simulink model "pso_mppt_grid_det"  (R2024a)
settings: Solver=FixedStepDiscrete  StartTime=0.0  StopTime=2.5  RelTol=1e-3
PreLoadFcn:
  | Ts_Power=1e-6;
  | Ts_Control=100e-6;
undefined symbols (not defined in the file or in its folder): D1, Delta, sigbuilder_block
libraries: spsSeriesRLCBranchLib x5, spsMeanLib x3, spsThreePhaseTransformerTwoWindingsLib x2, spsDistributedParametersLineLib x2, spsThreePhaseParallelRLCLoadLib x2, slpidlib x2, spsabctodq0Lib x2, spsVoltageMeasurementLib x2, spsPWMGeneratorDCDCLib x1, spsThreePhaseSeriesRLCLoadLib x1, spsThreeLevelBridgeLib x1, spsThreePhaseSourceLib x1
(part 1 of 2)
Description:
  | Copyright 2008-2019 The MathWorks, Inc.
settings Model: SimulationMode=accelerator  Creator=MathWorks  LastModifiedBy=Administrator
settings SolverCC: AlgebraicLoopSolver=TrustRegion
settings DataIOCC: LimitDataPoints=on  SaveFormat=Array  SignalLoggingSaveFormat=ModelDataLogs  SignalLogging=off  DSMLogging=off  ReturnWorkspaceOutputs=off
settings OptimizationCC: ExpressionDepthLimit=2147483647  LifeSpan=inf
settings DebuggingCC: UnderspecifiedInitializationDetection=Classic  MergeDetectMultiDrivingBlocksExec=none  SolverPrmCheckMsg=warning  FcnCallInpInsideContextMsg=warning  UnconnectedInputMsg=warning  UnconnectedOutputMsg=warning  UnconnectedLineMsg=warning  StateNameClashWarn=warning  SFUnexpectedBacktrackingDiag=warning  SFNoUnconditionalDefaultTransitionDiag=warning  SFExecutionAtInitializationDiag=none  ArithmeticOperatorsInVariantConditions=warning
settings HardwareCC: ProdBitPerPointer=32  ProdBitPerSizeT=32  ProdBitPerPtrDiffT=32  ProdLargestAtomicFloat=None  ProdIntDivRoundTo=Undefined  ProdEndianess=Unspecified  ProdWordSize=32  ProdHWDeviceType=32-bit Generic
settings ModelReferenceCC: EnableRefExpFcnMdlSchedulingChecks=on  PropagateSignalLabelsOutOfModel=off
settings SFSimCC: SimUseLocalCustomCode=off  CustomCodeUndefinedFunction=UseInterfaceOnly
settings RTWCC: RTWUseLocalCustomCode=off  GPUComputeCapability=3.5
settings CodeAppCC: StateflowObjectComments=on
settings GRTTargetCC: TargetLangStandard=C89/C90 (ANSI)  CombineOutputUpdateFcns=off  GRTInterface=on
settings ConfigComp: CovMetricSettings=dw  CovSaveCumulativeToWorkspaceVar=on  CovSaveSingleToWorkspaceVar=on  CovExternalEMLEnable=off  CovSFcnEnable=off
settings SimscapeCC: SimscapeNormalizeSystem=off

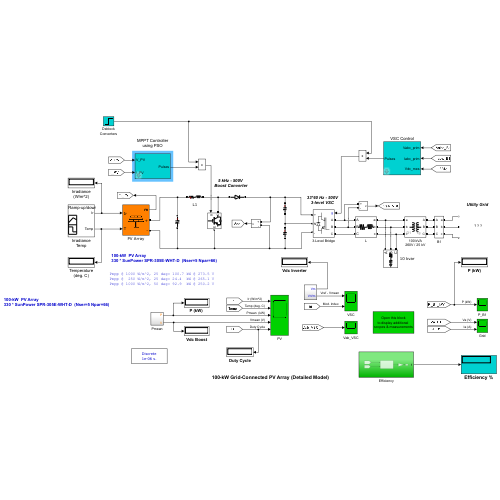
[thumbnail: Simulink's stored preview of the top-level diagram]
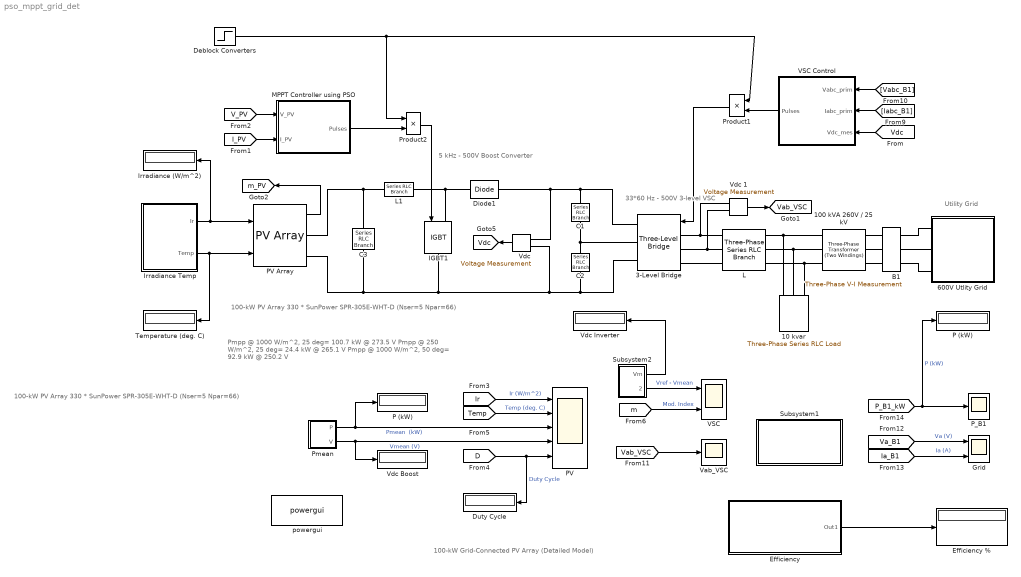
== system pso_mppt_grid_det ==
  note: 5 kHz - 500V
      | Boost Converter
  note: 33*60 Hz - 500V
      | 3-level VSC
  note: 100-kW Grid-Connected PV Array (Detailed Model)
  note: Utility Grid
  note: Pmpp @ 1000 W/m^2, 25 deg= 100.7 kW @ 273.5 V
      | Pmpp @  250 W/m^2, 25 deg= 24.4  kW @ 265.1 V
      | Pmpp @ 1000 W/m^2, 50 deg= 92.9  kW @ 250.2 V
  note: 100-kW  PV Array
      | 330 * SunPower SPR-305E-WHT-D  (Nser=5 Npar=66)
  note: 100-kW  PV Array
      | 330 * SunPower SPR-305E-WHT-D  (Nser=5 Npar=66)
  " MPPT Controller using PSO " : Subsystem  mask(Boost Control - MPPT){fc=5000, T_MPPT=200e-6, Dinit=0.5}
      mask prompts: fc "PWM switching frequency (Hz)"; T_MPPT "Time window used by MPPT control (s)"; Dinit "Initial value of duty cycle"
  10 kvar : spsThreePhaseSeriesRLCLoadLib/Three-Phase Series RLC Load  LConnTagsString=A|B|C  Configuration=Y (grounded)  NominalVoltage=240  Vabc=[1e3 1e3 1e3]  Vabcp=[1e3 1e3 1e3]  NominalFrequency=60  UnbalancedPower=off  ActivePower=10e3/100  InductivePower=0  CapacitivePower=10e3  Pabc=[10e3 9e3 11e3]  QLabc=[100 90 110]  QCabc=[100 90 110]  Pabcp=[10e3 9e3 11e3]  QLabcp=[100 90 110]  QCabcp=[100 90 110]  Measurements=None  LoadType=constant Z
  100 kVA 260V / 25 kV : spsThreePhaseTransformerTwoWindingsLib/Three-Phase Transformer (Two Windings)  Winding1Connection=Yg  Winding2Connection=Delta (D1)  CoreType=Three single-phase transformers  SetSaturation=off  Hysteresis=off  DataFile='hysteresis'  SetInitialFlux=off  Measurements=None  UNITS=pu  NominalPower=[100e3 , 60 ]  Winding1=[ 25e3 , 0.001 , 0.03 ]  Winding2=[ 260 , 0.001 , 0.03 ]  Rm=500  Lm=500  L0=0.5  Saturation=[ 0,0 ; 0.0024,1.2 ; 1.0,1.52 ]  InitialFluxes=[ 0.8 , -0.8 , 0.7 ]  BreakLoop=off  DiscreteSolver=Trapezoidal iterative  DataType=off  TransfoNumber=0
  3-Level Bridge : spsThreeLevelBridgeLib/Three-Level Bridge  Arms=3  SnubberResistance=1e6  SbubberCapacitance=inf  Device=IGBT / Diodes  Ron=0.2e-3  ForwardVoltages="[  0  0 ]"  Measurements=None
      settings: AttributesFormatString=\n  LibrarySourceBlock=sps_lib/Power Electronics/Three-Level Bridge
  600V Utlity Grid : Subsystem
      mask Display: image(imread('grid.jpg'))
  B1 : spsThreePhaseVIMeasurementLib/Three-Phase V-I Measurement  VoltageMeasurement=phase-to-ground  SetLabelV=on  LabelV=Vabc_B1  Vpu=off  VpuLL=off  CurrentMeasurement=yes  SetLabelI=on  LabelI=Iabc_B1  Ipu=off  Pbase=100e6  Vbase=500e3  OutputType=Magnitude  PhasorSimulation=off  PSBequivalent=0
  C1 : spsSeriesRLCBranchLib/Series RLC Branch  LConnTagsString=__new0  RConnTagsString=__new0  BranchType=C  Resistance=1.0  Inductance=1.0  SetiL0=off  InitialCurrent=0  Capacitance=12000e-06  Setx0=off  InitialVoltage=0  Measurements=None
  C2 : spsSeriesRLCBranchLib/Series RLC Branch  LConnTagsString=__new0  RConnTagsString=__new0  BranchType=C  Resistance=1.0  Inductance=1.0  SetiL0=off  InitialCurrent=0  Capacitance=12000e-06  Setx0=off  InitialVoltage=0  Measurements=None
  C3 : spsSeriesRLCBranchLib/Series RLC Branch  LConnTagsString=__new0  RConnTagsString=__new0  BranchType=C  Resistance=1.0  Inductance=1.0  SetiL0=off  InitialCurrent=0  Capacitance=100e-6  Setx0=off  InitialVoltage=0  Measurements=Branch voltage
  Deblock Converters : Step  Time=0.05  SampleTime=0
  Diode1 : spsDiodeLib/Diode  Ron=1e-4  Lon=0  Vf=0  IC=0  UseSnubber=off  Rs=inf  Cs=inf  Measurements=off
  Duty Cycle : Display
      settings: Format=bank  Decimation=2000
  Efficiency : Subsystem
  Efficiency % : Display
  Grid : Scope  NumInputPorts=2
  IGBT1 : spsIGBTLib/IGBT  Ron=0.001  Lon=0  Vf=0  Tf=0  Tt=0  IC=0  Rs=1e5  Cs=inf  Measurements=off
  Irradiance (W/m^2) : Display
      settings: Format=bank  Decimation=1000
  Irradiance Temp : Subsystem  Tag=STV Subsys  LoadFcn=sigbuilder_block('load');  StartFcn=sigbuilder_block('start');  StopFcn=sigbuilder_block('stop');  ClipboardFcn=sigbuilder_block('clipboard');  mask(Sigbuilder block){tuvar=[0:10]}
      mask help: Sigbuilder GUI
      mask init:
      | if ~strcmp(get_param(bdroot(gcbh),'SimulationStatus'),'stopped') tuvar = sigbuilder_block('maskInit'); end
      settings: CopyFcn=sigbuilder_block('copy');  DeleteFcn=sigbuilder_block('delete');  ModelCloseFcn=sigbuilder_block('modelClose');  PreSaveFcn=sigbuilder_block('preSave');  PauseFcn=sigbuilder_block('pause')  ContinueFcn=sigbuilder_block('continue')  NameChangeFcn=sigbuilder_block('namechange');  OpenFcn=sigbuilder_block('open',[216.75 153.75 550.5 395.25 ]);  CloseFcn=sigbuilder_block('close');
      mask Display: plot(0, 0, 100, 100,[2, 2, 32, 32, 2], [68, 8, 8, 68, 68],[32, 2], [38, 38], [32, 19, 2],[53, 60, 44], [32, 17, 17, 2],[16, 16, 31, 31]);txt = getActiveGroup(gcbh);text(2, 100, txt,'verticalAlignment', 'top');
  L : spsThreePhaseSeriesRLCBranchLib/Three-Phase Series RLC Branch  LConnTagsString=A|B|C  RConnTagsString=A|B|C  BranchType=RL  Resistance=500e-6*377/50/2  Inductance=500e-6/2  Capacitance=inf  Measurements=None
  L1 : spsSeriesRLCBranchLib/Series RLC Branch  LConnTagsString=__new0  RConnTagsString=__new0  BranchType=RL  Resistance=0.005  Inductance=5e-3  SetiL0=off  InitialCurrent=0  Capacitance=1e-6  Setx0=off  InitialVoltage=0  Measurements=None
  P (kW) : Display
      settings: Format=bank  Decimation=2000
  "P (kW) " : Display
      settings: Format=bank  Decimation=2000
  PV : Scope  NumInputPorts=5
  PV Array : spsPVArrayLib/PV Array  Npar=66  Nser=5  PlotType=array @ 1000 W/m2 & specified temperatures  S_vec="[ 1000  250 ]"  Temp_C_vec="[0 25 50  ]"  ModuleName=SunPower SPR-305E-WHT-D  PlotWhenSelected=off  Pm=305.226  Ncell=96  Voc=64.2  Isc=5.96  Vm=54.7  Im=5.58  beta_Voc_pc=-0.2727  alpha_Isc_pc=0.061745  beta_Voc=-0.17507  alpha_Isc=0.00368  IL=5.9657  I0=6.3076e-12  nI=0.94489  Rsh=393.2054  Rs=0.37428  RobustModel=off  RobustCellTemperature=313.3991  BAL=on  Tc=Tc  Tfilter=5e-5
  P_B1 : Scope
  Pmean : Subsystem
  Product1 : Product  RndMeth=Zero
  Product2 : Product  RndMeth=Zero
  Subsystem1 : Subsystem
      mask Display: disp('Open this block\nto display additional \nscopes & measurements')
  Subsystem2 : Subsystem
  Temperature (deg. C) : Display
      settings: Format=bank  Decimation=1000
  VSC : Scope  NumInputPorts=2
  VSC Control : Subsystem  mask(VSC Main Controller){nom=[ 100e3  60 ], Vnom=[ 25e3 260 ], Vnom_dc=500, RLxfo=[0.002  0.06 ], RLchoke=[2e-3  250e-6  ], K_VDCreg=[7  800], K_Ireg=[0.3 20], Ts=Ts_Control}
      mask prompts: nom "Nominal power and frequency [ Pnom(VA)  Fnom(Hz) ]:"; Vnom "Nominal primary and secondary voltages (Vrms LL) [ Vnom_prim   Vnom_sec ]:"; Vnom_dc "Nominal DC bus voltage (V):"; RLxfo "Total transformer leakage impedance (pu/Pnom) [ Rxfo  Lxf ]"; RLchoke "Choke impedance [ R(ohm) L(H) ]"; K_VDCreg "VDC regultator gains [ Kp  Ki ]:"; K_Ireg "Current regulator gains [ Kp  Ki ]:"; Ts "Sample time"
      mask init:
      | Pnom=nom(1);
      | Fnom=nom(2);
      | Vnom_prim=Vnom(1);
      | Vnom_sec=Vnom(2);
      | Zbase=Vnom_sec^2/Pnom;
      | Rtot_pu=RLxfo(1) + RLchoke(1)/Zbase;
      | Ltot_pu=RLxfo(2) + RLchoke(2)/(Zbase/(2*pi*Fnom));
      | Kp_VDCreg=K_VDCreg(1);
      | Ki_VDCreg=K_VDCreg(2);
      | Kp_Ireg=K_Ireg(1);
      | Ki_Ireg=K_Ireg(2);
      | Vdc_ref=Vnom_dc;
      | % Used to determine initial value of Boost Control (MPPT)
      | assignin('base','Vdc_ref_Inv',Vdc_ref);
  Vab_VSC : Scope
  "Vdc " : spsVoltageMeasurementLib/Voltage Measurement  Tag=PoWeRsYsTeMmEaSuReMeNt  PhasorSimulation=off  OutputType=Magnitude  PSBequivalent=0
  Vdc 1 : spsVoltageMeasurementLib/Voltage Measurement  Tag=PoWeRsYsTeMmEaSuReMeNt  PhasorSimulation=off  OutputType=Magnitude  PSBequivalent=0
  Vdc Boost : Display
      settings: Format=bank  Decimation=2000
  Vdc Inverter : Display
      settings: Format=bank  Decimation=2000
  powergui : spspowerguiLib/powergui  Priority=1  SimulationMode=Discrete  SampleTime=Ts_Power  frequency=60  Iterations=50  frequencyindice=0  Pbase=100e6  ErrMax=1e-4  UnitsV=kV  UnitsW=MW  buscounter=0  FunctionMessages=off  echomessages=off  EnableUseOfTLC=off  CurrentSourceSwitches=off  DisableSnubberDevices=off  DisableRonSwitches=off  DisableVfSwitches=off  DisplayEquations=off  AutomaticDiscreteSolvers=off  SolverType=Tustin/Backward Euler (TBE)  Interpol=off  ExternalGateDelay=off  methode=off  Ts=0  x0status=blocks  SPID=off  SwTol=0  HookPort=off  NonlinearTolerance=0  nMaxIteration=15  ContinueOnMaxIteration=off  RestoreLinks=warning  ResistiveCurrentMeasurement=off  Frange=[0:2:500]  Ylog=off  Xlog=on  ShowGrid=off  save=off  variable=ZData  structure=0  ZoomFFT=on  StartTime=0.0  cycles=1  DisplayStyle=1  fundamental=60  FreqAxis=off  MaxFrequency=1000  frequencyindicesteady=1  RmsSteady=1  display=off
  tag scope: Vab_VSC=global, Vdc=global, m_PV=global
  wires:
  "Vdc "/1 -> [Vdc]
  Product2/1 -> IGBT1/1
  " MPPT Controller using PSO "/1(Pulses) -> Product2/2
  Deblock Converters/1 -> Product2/1, Product1/1
  [Vabc_B1] -> VSC Control/1(Vabc_prim)
  [Iabc_B1] -> VSC Control/2(Iabc_prim)
  [Vdc] -> VSC Control/3(Vdc_mes)
  VSC Control/1(Pulses) -> Product1/2
  Product1/1 -> 3-Level Bridge/1
  [I_PV] -> " MPPT Controller using PSO "/2(I_PV)
  [V_PV] -> " MPPT Controller using PSO "/1(V_PV)
  Pmean/1(P) -> "P (kW) "/1, PV/3  "Pmean  (kW)"
  [m] -> VSC/2  "Mod. Index"
  Vdc 1/1 -> [Vab_VSC]
  [Vab_VSC] -> Vab_VSC/1
  [Ia_B1] -> Grid/2  "Ia (A)"
  [Va_B1] -> Grid/1  "Va (V)"
  [P_B1_kW] -> P_B1/1, P (kW)/1  "P (kW)"
  Pmean/2(V) -> Vdc Boost/1, PV/4  "Vmean (V)"
  Subsystem2/2(VrVm) -> VSC/1  "Vref - Vmean"
  Subsystem2/1(Vm) -> Vdc Inverter/1
  PV Array/1 -> [m_PV]
  Irradiance Temp/1(Ir) -> PV Array/1, Irradiance (W/m^2)/1
  Irradiance Temp/2(Temp) -> PV Array/2, Temperature (deg. C)/1
  [D] -> Duty Cycle/1, PV/5  "Duty Cycle"
  [Temp] -> PV/2  "Temp (deg. C)"
  [Ir] -> PV/1  "Ir (W/m^2)"
  Efficiency/1(Out1) -> Efficiency %/1
  connections:
  3-Level Bridge/RConn1 -- Diode1/RConn1 -- "Vdc "/LConn1 -- C1/LConn1
  L1/RConn1 -- Diode1/LConn1 -- IGBT1/LConn1
  3-Level Bridge/RConn3 -- C2/RConn1 -- "Vdc "/LConn2 -- IGBT1/RConn1 -- PV Array/RConn2 -- C3/RConn1
  3-Level Bridge/LConn1 -- L/LConn1 -- Vdc 1/LConn1
  3-Level Bridge/LConn2 -- L/LConn2 -- Vdc 1/LConn2
  3-Level Bridge/LConn3 -- L/LConn3
  L/RConn1 -- 100 kVA 260V / 25 kV/RConn1 -- 10 kvar/LConn1
  L/RConn2 -- 100 kVA 260V / 25 kV/RConn2 -- 10 kvar/LConn2
  L/RConn3 -- 100 kVA 260V / 25 kV/RConn3 -- 10 kvar/LConn3
  B1/LConn1 -- 100 kVA 260V / 25 kV/LConn1
  B1/LConn2 -- 100 kVA 260V / 25 kV/LConn2
  B1/LConn3 -- 100 kVA 260V / 25 kV/LConn3
  C2/LConn1 -- C1/RConn1 -- 3-Level Bridge/RConn2
  C3/LConn1 -- PV Array/RConn1 -- L1/LConn1
  B1/RConn2 -- 600V Utlity Grid/LConn2
  B1/RConn1 -- 600V Utlity Grid/LConn1
  B1/RConn3 -- 600V Utlity Grid/LConn3

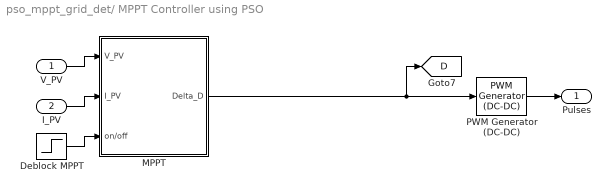
== system pso_mppt_grid_det/ MPPT Controller using PSO  ==
  V_PV : Inport
  I_PV : Inport  Port=2
  Deblock MPPT : Step  Time=0.4  SampleTime=0
  MPPT : Subsystem
  PWM Generator (DC-DC) : spsPWMGeneratorDCDCLib/PWM Generator (DC-DC)  Fsw=fc  Ts=Ts_Power
  Pulses : Outport  VectorParamsAs1DForOutWhenUnconnected=off
  tag scope: D=global
  wires:
  V_PV/1 -> MPPT/1(V_PV)
  I_PV/1 -> MPPT/2(I_PV)
  PWM Generator (DC-DC)/1 -> Pulses/1
  Deblock MPPT/1 -> MPPT/3(on/off)
  MPPT/1(Delta_D) -> PWM Generator (DC-DC)/1, [D]

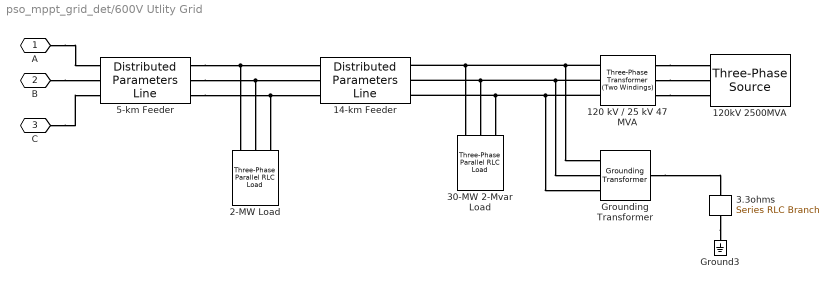
== system pso_mppt_grid_det/600V Utlity Grid ==
  120 kV / 25 kV 47 MVA : spsThreePhaseTransformerTwoWindingsLib/Three-Phase Transformer (Two Windings)  Winding1Connection=Yg  Winding2Connection=Delta (D1)  CoreType=Three single-phase transformers  SetSaturation=off  Hysteresis=off  DataFile='basic_model'  SetInitialFlux=off  Measurements=None  UNITS=pu  NominalPower=[47e6 60 ]  Winding1="[ 120e3  0.08/30   0.08 ]"  Winding2="[ 25e3  0.08/30  0.08]"  Rm=500  Lm=500  L0=0.5  Saturation="[ 0,0  ;  0.005,1.2  ;  1.0,1.4 ]"  InitialFluxes=[ 0.8 , -0.8 , 0.7 ]  BreakLoop=off  DiscreteSolver=Trapezoidal iterative  DataType=off  TransfoNumber=0
  120kV 2500MVA : spsThreePhaseSourceLib/Three-Phase Source  InternalConnection=Yg  VoltagePhases=off  Voltage=120e3  PhaseAngle=0  Voltage_phases=[25e3 25e3 25e3]/sqrt(3)  PhaseAngles_phases=[0 -120 +120]  Frequency=60  NonIdealSource=on  SpecifyImpedance=on  Resistance=0.8929  Inductance=16.58e-3  ShortCircuitLevel=2500e6  BaseVoltage=120e3  XRratio=7  BusType=swing  Pref=0  Qref=0  Prefabc=[10e3, 10e3, 10e3]  Qrefabc=[0, 0, 0]  Qmin=-inf  Qmax=inf
  14-km Feeder : spsDistributedParametersLineLib/Distributed Parameters Line  Phases=3  Length=14  Frequency=60  Resistance=[0.1153 0.413]  Inductance=[1.05e-3 3.32e-3]  Capacitance=[11.33e-009 5.01e-009]  x1=[-5.8e-05 -1.56321761301392e-09 0 0;-5.7e-05 -1.56319609439298e-09 0 0;-5.6e-05 -1.56317435360702e-09 0 0;-5.5e-05 -1.56315239065911e-09 0 0;-5.4e-05 -1.5631302055524e-09 0 0;-5.3e-05 -1.56310779829001e-09 0 0;-5.2e-05 -1.56308516887515e-09 0 0;-5.1e-05 -1.56306231731103e-09 0 0;-5e-05 -1.5630392436009e-09 0 0;-4.9e-05 -1.56301594774803e-09 -3790.73535190163 -24061.4134200248;-4.8e-05 -1.56299242975573e-09 -3781.66414358624 -24062.8407837192;-4.7e-05 -1.56296868962735e-09 -3772.59239781203 -24064.2647275473;-4.6e-05 -1.56294472736627e-09 -3763.52011586831 -24065.6852513067;-4.5e-05 -1.56292054297588e-09 -3754.44729904445 -24067.1023547955;-4.4e-05 -1.56289613645963e-09 -3745.37394862989 -24068.5160378124;-4.3e-05 -1.56287150782099e-09 -3736.30006591417 -24069.9263001563;-4.2e-05 -1.56284665706344e-09 -3727.22565218688 -24071.3331416269;-4.1e-05 -1.56282158419054e-09 -3718.15070873771 -24072.7365620243;-4e-05 -1.56279628920583e-09 -3709.0752368564 -24074.1365611489;-3.9e-05 -1.56277077211291e-09 -3699.99923783278 -24075.5331388018;-3.8e-05 -1.56274503291542e-09 -3690.92271295675 -24076.9262947845;-3.7e-05 -1.56271907161701e-09 -3681.84566351829 -24078.3160288991;-3.6e-05 -1.56269288822136e-09 -3672.76809080744 -24079.7023409479;-3.5e-05 -1.56266648273221e-09 -3663.68999611435 -24081.085230734;-3.4e-05 -1.56263985515329e-09 -3654.6113807292 -24082.4646980609;-3.3e-05 -1.56261300548841e-09 -3645.53224594227 -24083.8407427325;-3.2e-05 -1.56258593374137e-09 -3636.4525930439 -24085.2133645531;-3.1e-05 -1.56255863991601e-09 -3627.37242332452 -24086.5825633279;-3e-05 -1.56253112401623e-09 -3618.29173807463 -24087.948338862;-2.9e-05 -1.56250338604593e-09 -3609.21053858478 -24089.3106909615;-2.8e-05 -1.56247542600905e-09 -3600.12882614563 -24090.6696194327;-2.7e-05 -1.56244724390957e-09 -3591.04660204788 -24092.0251240825;-2.6e-05 -1.56241883975148e-09 -3581.96386758232 -24093.3772047183;-2.5e-05 -1.56239021353884e-09 -3572.88062403981 -24094.7258611478;-2.4e-05 -1.5623613652757e-09 -3563.79687271129 -24096.0710931794;-2.3e-05 -1.56233229496617e-09 -3554.71261488775 -24097.412900622;-2.2e-05 -1.56230300261438e-09 -3545.62785186027 -24098.7512832847;-2.1e-05 -1.56227348822449e-09 -3536.54258492 -24100.0862409775;-2e-05 -1.56224375180069e-09 -3527.45681535816 -24101.4177735105;-1.9e-05 -1.56221379334722e-09 -3518.37054446603 -24102.7458806945;-1.8e-05 -1.56218361286833e-09 -3509.28377353499 -24104.0705623409;-1.7e-05 -1.5621532103683e-09 -3500.19650385646 -24105.3918182612;-1.6e-05 -1.56212258585147e-09 -3491.10873672194 -24106.7096482678;-1.5e-05 -1.56209173932218e-09 -3482.02047342302 -24108.0240521733;-1.4e-05 -1.56206067078481e-09 -3472.93171525133 -24109.3350297909;-1.3e-05 -1.56202938024379e-09 -3463.84246349859 -24110.6425809344;-1.2e-05 -1.56199786770356e-09 -3454.75271945659 -24111.9467054178;-1.1e-05 -1.56196613316859e-09 -3445.66248441718 -24113.2474030559;-1e-05 -1.5619341766434e-09 -3436.57175967229 -24114.5446736637;-9e-06 -1.56190199813254e-09 -3427.48054651391 -24115.838517057;-8e-06 -1.56186959764056e-09 -3418.38884623411 -24117.1289330518;-7e-06 -1.56183697517209e-09 -3409.29666012501 -24118.4159214647;-6e-06 -1.56180413073174e-09 -3400.20398947883 -24119.6994821128;-5e-06 -1.5617710643242e-09 -3391.11083558782 -24120.9796148137;-4e-06 -1.56173777595416e-09 -3382.01719974435 -24122.2563193855;-3e-06 -1.56170426562636e-09 -3372.9230832408 -24123.5295956467;-2e-06 -1.56167053334555e-09 -3363.82848736966 -24124.7994434163;-1e-06 -1.56163657911652e-09 -3354.73341342347 -24126.0658625139]  x2=[-5.8e-05 -1.66978294033676e-09 0 0;-5.7e-05 -1.6697278258948e-09 0 0;-5.6e-05 -1.66967247414727e-09 0 0;-5.5e-05 -1.66961688510205e-09 0 0;-5.4e-05 -1.66956105876704e-09 0 0;-5.3e-05 -1.66950499515017e-09 0 0;-5.2e-05 -1.6694486942594e-09 0 0;-5.1e-05 -1.66939215610274e-09 0 0;-5e-05 -1.66933538068823e-09 0 0;-4.9e-05 -1.66927836802393e-09 -3379.39242591515 -24244.0512732149;-4.8e-05 -1.66922111811794e-09 -3370.25239398334 -24245.3235513048;-4.7e-05 -1.66916363097841e-09 -3361.11188306351 -24246.5923835935;-4.6e-05 -1.6691059066135e-09 -3351.97089445472 -24247.8577699007;-4.5e-05 -1.66904794503142e-09 -3342.82942945612 -24249.1197100465;-4.4e-05 -1.6689897462404e-09 -3333.6874893669 -24250.3782038516;-4.3e-05 -1.66893131024872e-09 -3324.54507548634 -24251.6332511372;-4.2e-05 -1.66887263706468e-09 -3315.40218911378 -24252.8848517248;-4.1e-05 -1.66881372669662e-09 -3306.25883154863 -24254.1330054366;-4e-05 -1.66875457915291e-09 -3297.11500409037 -24255.3777120952;-3.9e-05 -1.66869519444196e-09 -3287.97070803853 -24256.6189715237;-3.8e-05 -1.66863557257221e-09 -3278.82594469273 -24257.8567835457;-3.7e-05 -1.66857571355213e-09 -3269.68071535264 -24259.0911479852;-3.6e-05 -1.66851561739023e-09 -3260.535021318 -24260.3220646668;-3.5e-05 -1.66845528409505e-09 -3251.38886388862 -24261.5495334157;-3.4e-05 -1.66839471367516e-09 -3242.24224436437 -24262.7735540573;-3.3e-05 -1.66833390613917e-09 -3233.09516404519 -24263.9941264176;-3.2e-05 -1.66827286149574e-09 -3223.94762423108 -24265.2112503233;-3.1e-05 -1.66821157975352e-09 -3214.79962622212 -24266.4249256013;-3e-05 -1.66815006092123e-09 -3205.65117131843 -24267.6351520791;-2.9e-05 -1.66808830500762e-09 -3196.50226082022 -24268.8419295848;-2.8e-05 -1.66802631202146e-09 -3187.35289602775 -24270.0452579468;-2.7e-05 -1.66796408197155e-09 -3178.20307824136 -24271.2451369941;-2.6e-05 -1.66790161486676e-09 -3169.05280876142 -24272.4415665561;-2.5e-05 -1.66783891071595e-09 -3159.90208888841 -24273.6345464629;-2.4e-05 -1.66777596952803e-09 -3150.75091992283 -24274.8240765449;-2.3e-05 -1.66771279131195e-09 -3141.59930316529 -24276.010156633;-2.2e-05 -1.6676493760767e-09 -3132.44723991642 -24277.1927865587;-2.1e-05 -1.66758572383127e-09 -3123.29473147694 -24278.3719661539;-2e-05 -1.66752183458473e-09 -3114.14177914762 -24279.547695251;-1.9e-05 -1.66745770834614e-09 -3104.98838422931 -24280.7199736828;-1.8e-05 -1.66739334512462e-09 -3095.8345480229 -24281.8888012829;-1.7e-05 -1.66732874492933e-09 -3086.68027182936 -24283.054177885;-1.6e-05 -1.66726390776943e-09 -3077.52555694971 -24284.2161033236;-1.5e-05 -1.66719883365416e-09 -3068.37040468505 -24285.3745774335;-1.4e-05 -1.66713352259274e-09 -3059.21481633652 -24286.52960005;-1.3e-05 -1.66706797459448e-09 -3050.05879320534 -24287.6811710091;-1.2e-05 -1.66700218966867e-09 -3040.90233659279 -24288.829290147;-1.1e-05 -1.66693616782468e-09 -3031.7454478002 -24289.9739573006;-1e-05 -1.66686990907188e-09 -3022.58812812896 -24291.1151723072;-9e-06 -1.6668034134197e-09 -3013.43037888055 -24292.2529350046;-8e-06 -1.66673668087757e-09 -3004.27220135647 -24293.387245231;-7e-06 -1.666669711455e-09 -2995.11359685831 -24294.5181028254;-6e-06 -1.66660250516148e-09 -2985.95456668772 -24295.645507627;-5e-06 -1.66653506200659e-09 -2976.79511214638 -24296.7694594754;-4e-06 -1.66646738199989e-09 -2967.63523453608 -24297.8899582111;-3e-06 -1.66639946515102e-09 -2958.47493515863 -24299.0070036747;-2e-06 -1.66633131146961e-09 -2949.3142153159 -24300.1205957076;-1e-06 -1.66626292096537e-09 -2940.15307630986 -24301.2307341513]  x3=[-5.8e-05 -7.7854813363112e-12 0 0;-5.7e-05 -7.78653747717526e-12 0 0;-5.6e-05 -7.78759251139869e-12 0 0;-5.5e-05 -7.78864643883155e-12 0 0;-5.4e-05 -7.78969925932404e-12 0 0;-5.3e-05 -7.79075097272655e-12 0 0;-5.2e-05 -7.7918015788896e-12 0 0;-5.1e-05 -7.79285107766388e-12 0 0;-5e-05 -7.79389946890022e-12 0 0;-4.9e-05 -7.79494675244963e-12 -23.5442847382768 -155.68147777382;-4.8e-05 -7.79599292816327e-12 -23.4855925321581 -155.690342696941;-4.7e-05 -7.79703799589245e-12 -23.426896988213 -155.699185492992;-4.6e-05 -7.79808195548864e-12 -23.3681981147833 -155.708006160717;-4.5e-05 -7.79912480680348e-12 -23.3094959202115 -155.716804698861;-4.4e-05 -7.80016654968874e-12 -23.2507904128405 -155.725581106174;-4.3e-05 -7.80120718399639e-12 -23.1920816010137 -155.73433538141;-4.2e-05 -7.80224670957851e-12 -23.1333694930749 -155.743067523323;-4.1e-05 -7.80328512628737e-12 -23.0746540973683 -155.751777530673;-4e-05 -7.80432243397539e-12 -23.0159354222388 -155.760465402222;-3.9e-05 -7.80535863249514e-12 -22.9572134760315 -155.769131136735;-3.8e-05 -7.80639372169936e-12 -22.8984882670923 -155.777774732981;-3.7e-05 -7.80742770144093e-12 -22.8397598037672 -155.786396189731;-3.6e-05 -7.80846057157291e-12 -22.7810280944028 -155.794995505759;-3.5e-05 -7.8094923319485e-12 -22.7222931473463 -155.803572679844;-3.4e-05 -7.81052298242106e-12 -22.6635549709452 -155.812127710767;-3.3e-05 -7.81155252284412e-12 -22.6048135735475 -155.820660597312;-3.2e-05 -7.81258095307136e-12 -22.5460689635017 -155.829171338265;-3.1e-05 -7.81360827295661e-12 -22.4873211491567 -155.837659932419;-3e-05 -7.81463448235386e-12 -22.4285701388618 -155.846126378565;-2.9e-05 -7.81565958111728e-12 -22.3698159409669 -155.854570675501;-2.8e-05 -7.81668356910117e-12 -22.3110585638222 -155.862992822027;-2.7e-05 -7.81770644616e-12 -22.2522980157786 -155.871392816945;-2.6e-05 -7.81872821214839e-12 -22.1935343051872 -155.879770659062;-2.5e-05 -7.81974886692113e-12 -22.1347674403996 -155.888126347188;-2.4e-05 -7.82076841033317e-12 -22.0759974297679 -155.896459880134;-2.3e-05 -7.8217868422396e-12 -22.0172242816446 -155.904771256717;-2.2e-05 -7.82280416249568e-12 -21.9584480043827 -155.913060475754;-2.1e-05 -7.82382037095682e-12 -21.8996686063357 -155.921327536069;-2e-05 -7.82483546747861e-12 -21.8408860958573 -155.929572436485;-1.9e-05 -7.82584945191677e-12 -21.782100481302 -155.937795175832;-1.8e-05 -7.82686232412719e-12 -21.7233117710244 -155.945995752941;-1.7e-05 -7.82787408396593e-12 -21.6645199733797 -155.954174166645;-1.6e-05 -7.82888473128918e-12 -21.6057250967236 -155.962330415784;-1.5e-05 -7.82989426595331e-12 -21.5469271494121 -155.970464499197;-1.4e-05 -7.83090268781485e-12 -21.4881261398017 -155.978576415729;-1.3e-05 -7.83190999673048e-12 -21.4293220762493 -155.986666164226;-1.2e-05 -7.83291619255703e-12 -21.3705149671124 -155.994733743539;-1.1e-05 -7.8339212751515e-12 -21.3117048207488 -156.002779152522;-1e-05 -7.83492524437105e-12 -21.2528916455165 -156.010802390031;-9e-06 -7.83592810007299e-12 -21.1940754497744 -156.018803454925;-8e-06 -7.83692984211479e-12 -21.1352562418815 -156.026782346068;-7e-06 -7.83793047035408e-12 -21.0764340301974 -156.034739062326;-6e-06 -7.83892998464866e-12 -21.0176088230819 -156.042673602567;-5e-06 -7.83992838485646e-12 -20.9587806288955 -156.050585965664;-4e-06 -7.8409256708356e-12 -20.899949455999 -156.058476150493;-3e-06 -7.84192184244433e-12 -20.8411153127535 -156.066344155932;-2e-06 -7.84291689954108e-12 -20.7822782075207 -156.074189980863;-1e-06 -7.84391084198443e-12 -20.7234381486628 -156.082013624171]  x4=[-5.8e-05 4.3627087018527e-12 0 0;-5.7e-05 4.3644706519158e-12 0 0;-5.6e-05 4.36623198169028e-12 0 0;-5.5e-05 4.36799269092582e-12 0 0;-5.4e-05 4.36975277937219e-12 0 0;-5.3e-05 4.37151224677923e-12 0 0;-5.2e-05 4.3732710928969e-12 0 0;-5.1e-05 4.37502931747521e-12 0 0;-5e-05 4.37678692026428e-12 0 0;-4.9e-05 4.37854390101432e-12 -1.35581366009309 -2.15298522698308;-4.8e-05 4.38030025947562e-12 -1.35500190745795 -2.15349620368547;-4.7e-05 4.38205599539857e-12 -1.35418996224682 -2.15400687432802;-4.6e-05 4.38381110853364e-12 -1.3533778245751 -2.15451723883815;-4.5e-05 4.38556559863138e-12 -1.35256549455821 -2.15502729714334;-4.4e-05 4.38731946544244e-12 -1.3517529723116 -2.15553704917109;-4.3e-05 4.38907270871756e-12 -1.35094025795074 -2.15604649484895;-4.2e-05 4.39082532820757e-12 -1.35012735159114 -2.15655563410452;-4.1e-05 4.39257732366337e-12 -1.34931425334834 -2.15706446686544;-4e-05 4.39432869483598e-12 -1.34850096333789 -2.15757299305939;-3.9e-05 4.39607944147648e-12 -1.34768748167537 -2.1580812126141;-3.8e-05 4.39782956333604e-12 -1.34687380847641 -2.15858912545735;-3.7e-05 4.39957906016595e-12 -1.34605994385665 -2.15909673151694;-3.6e-05 4.40132793171756e-12 -1.34524588793175 -2.15960403072073;-3.5e-05 4.4030761777423e-12 -1.3444316408174 -2.16011102299662;-3.4e-05 4.40482379799173e-12 -1.34361720262934 -2.16061770827257;-3.3e-05 4.40657079221747e-12 -1.34280257348331 -2.16112408647655;-3.2e-05 4.40831716017121e-12 -1.34198775349508 -2.16163015753661;-3.1e-05 4.41006290160478e-12 -1.34117274278047 -2.16213592138081;-3e-05 4.41180801627006e-12 -1.3403575414553 -2.16264137793728;-2.9e-05 4.41355250391902e-12 -1.33954214963543 -2.16314652713417;-2.8e-05 4.41529636430375e-12 -1.33872656743675 -2.16365136889971;-2.7e-05 4.41703959717639e-12 -1.33791079497516 -2.16415590316213;-2.6e-05 4.4187822022892e-12 -1.33709483236662 -2.16466012984973;-2.5e-05 4.42052417939451e-12 -1.33627867972707 -2.16516404889085;-2.4e-05 4.42226552824476e-12 -1.33546233717253 -2.16566766021388;-2.3e-05 4.42400624859244e-12 -1.33464580481901 -2.16617096374723;-2.2e-05 4.42574634019018e-12 -1.33382908278255 -2.16667395941938;-2.1e-05 4.42748580279066e-12 -1.33301217117923 -2.16717664715884;-2e-05 4.42922463614666e-12 -1.33219507012516 -2.16767902689416;-1.9e-05 4.43096284001107e-12 -1.33137777973645 -2.16818109855396;-1.8e-05 4.43270041413683e-12 -1.33056030012928 -2.16868286206686;-1.7e-05 4.43443735827702e-12 -1.3297426314198 -2.16918431736157;-1.6e-05 4.43617367218475e-12 -1.32892477372425 -2.1696854643668;-1.5e-05 4.43790935561328e-12 -1.32810672715885 -2.17018630301135;-1.4e-05 4.43964440831591e-12 -1.32728849183986 -2.17068683322402;-1.3e-05 4.44137883004606e-12 -1.32647006788358 -2.17118705493368;-1.2e-05 4.44311262055723e-12 -1.32565145540631 -2.17168696806924;-1.1e-05 4.44484577960301e-12 -1.32483265452442 -2.17218657255965;-1e-05 4.44657830693707e-12 -1.32401366535425 -2.17268586833391;-9e-06 4.44831020231319e-12 -1.32319448801222 -2.17318485532105;-8e-06 4.45004146548523e-12 -1.32237512261474 -2.17368353345015;-7e-06 4.45177209620713e-12 -1.32155556927826 -2.17418190265035;-6e-06 4.45350209423293e-12 -1.32073582811927 -2.17467996285081;-5e-06 4.45523145931677e-12 -1.31991589925425 -2.17517771398075;-4e-06 4.45696019121285e-12 -1.31909578279976 -2.17567515596943;-3e-06 4.4586882896755e-12 -1.31827547887233 -2.17617228874615;-2e-06 4.4604157544591e-12 -1.31745498758856 -2.17666911224025;-1e-06 4.46214258531815e-12 -1.31663430906505 -2.17716562638113]  x5=5.70973484498186e-05  V1=ones(3,3)  V2=ones(3,3)  I1=ones(3,3)  I2=ones(3,3)  nHarmo=1  Measurements=None  Decoupling=off  VsMag0=0  VrMag0=0  VsAngle0=0  VrAngle0=0  IsMag0=0  IrMag0=0  IsAngle0=0  IrAngle0=0
      settings: LibrarySourceBlock=sps_lib/Power Grid Elements/Distributed Parameters Line
  2-MW Load : spsThreePhaseParallelRLCLoadLib/Three-Phase Parallel RLC Load  LConnTagsString=A|B|C  Configuration=Y (grounded)  NominalVoltage=25e3  Vabc=[1e3 1e3 1e3]  Vabcp=[1e3 1e3 1e3]  NominalFrequency=60  UnbalancedPower=off  ActivePower=2e6  InductivePower=0  CapacitivePower=0  Pabc=[10e3 9e3 11e3]  QLabc=[100 90 110]  QCabc=[100 90 110]  Pabcp=[10e3 9e3 11e3]  QLabcp=[100 90 110]  QCabcp=[100 90 110]  Measurements=None  LoadType=constant Z
  "3.3ohms " : spsSeriesRLCBranchLib/Series RLC Branch  LConnTagsString=__new0  RConnTagsString=__new0  BranchType=R  Resistance=3.3  Inductance=[]  SetiL0=off  InitialCurrent=0  Capacitance=[]  Setx0=off  InitialVoltage=0  Measurements=None
  30-MW 2-Mvar Load : spsThreePhaseParallelRLCLoadLib/Three-Phase Parallel RLC Load  LConnTagsString=A|B|C  Configuration=Y (grounded)  NominalVoltage=25e3  Vabc=[1e3 1e3 1e3]  Vabcp=[1e3 1e3 1e3]  NominalFrequency=60  UnbalancedPower=off  ActivePower=30e6  InductivePower=2e6  CapacitivePower=0  Pabc=[10e3 9e3 11e3]  QLabc=[100 90 110]  QCabc=[100 90 110]  Pabcp=[10e3 9e3 11e3]  QLabcp=[100 90 110]  QCabcp=[100 90 110]  Measurements=None  LoadType=constant Z
  5-km Feeder : spsDistributedParametersLineLib/Distributed Parameters Line  Phases=3  Length=5  Frequency=60  Resistance=[0.1153 0.413]  Inductance=[1.05e-3 3.32e-3]  Capacitance=[11.33e-009 5.01e-009]  x1=[-2.1e-05 -1.53861296656972e-09 -3537.17773129824 -24101.4118174687;-2e-05 -1.53858384697367e-09 -3528.09146196071 -24102.7435893521;-1.9e-05 -1.53855450871055e-09 -3519.00469120271 -24104.071935698;-1.8e-05 -1.53852495178452e-09 -3509.91742031565 -24105.3968563178;-1.7e-05 -1.53849517619978e-09 -3500.82965059105 -24106.7183510231;-1.6e-05 -1.53846518196056e-09 -3491.74138332049 -24108.0364196261;-1.5e-05 -1.53843496907113e-09 -3482.6526197956 -24109.3510619395;-1.4e-05 -1.53840453753579e-09 -3473.56336130811 -24110.6622777764;-1.3e-05 -1.53837388735885e-09 -3464.4736091498 -24111.9700669505;-1.2e-05 -1.53834301854467e-09 -3455.38336461252 -24113.2744292759;-1.1e-05 -1.53831193109764e-09 -3446.29262898821 -24114.5753645672;-1e-05 -1.53828062502218e-09 -3437.20140356885 -24115.8728726396;-9e-06 -1.53824910032274e-09 -3428.10968964652 -24117.1669533086;-8e-06 -1.53821735700379e-09 -3419.01748851335 -24118.4576063904;-7e-06 -1.53818539506986e-09 -3409.92480146155 -24119.7448317014;-6e-06 -1.53815321452547e-09 -3400.83162978339 -24121.0286290588;-5e-06 -1.53812081537521e-09 -3391.7379747712 -24122.3089982801;-4e-06 -1.53808819762368e-09 -3382.64383771741 -24123.5859391833;-3e-06 -1.53805536127551e-09 -3373.54921991449 -24124.8594515869;-2e-06 -1.53802230633537e-09 -3364.45412265499 -24126.12953531;-1e-06 -1.53798903280797e-09 -3355.35854723153 -24127.3961901721]  x2=[-2.1e-05 -1.56136582208046e-09 -3536.54258492 -24100.0862409775;-2e-05 -1.56133599729157e-09 -3527.45681535816 -24101.4177735105;-1.9e-05 -1.56130595060202e-09 -3518.37054446603 -24102.7458806945;-1.8e-05 -1.56127568201608e-09 -3509.28377353499 -24104.0705623409;-1.7e-05 -1.56124519153804e-09 -3500.19650385646 -24105.3918182612;-1.6e-05 -1.56121447917224e-09 -3491.10873672194 -24106.7096482678;-1.5e-05 -1.56118354492305e-09 -3482.02047342302 -24108.0240521733;-1.4e-05 -1.56115238879486e-09 -3472.93171525133 -24109.3350297909;-1.3e-05 -1.56112101079209e-09 -3463.84246349859 -24110.6425809344;-1.2e-05 -1.56108941091922e-09 -3454.75271945659 -24111.9467054178;-1.1e-05 -1.56105758918072e-09 -3445.66248441718 -24113.2474030559;-1e-05 -1.56102554558113e-09 -3436.57175967229 -24114.5446736637;-9e-06 -1.56099328012499e-09 -3427.48054651391 -24115.838517057;-8e-06 -1.5609607928169e-09 -3418.38884623411 -24117.1289330518;-7e-06 -1.56092808366147e-09 -3409.29666012501 -24118.4159214647;-6e-06 -1.56089515266334e-09 -3400.20398947883 -24119.6994821128;-5e-06 -1.5608619998272e-09 -3391.11083558782 -24120.9796148137;-4e-06 -1.56082862515776e-09 -3382.01719974435 -24122.2563193855;-3e-06 -1.56079502865977e-09 -3372.9230832408 -24123.5295956467;-2e-06 -1.56076121033799e-09 -3363.82848736966 -24124.7994434163;-1e-06 -1.56072717019724e-09 -3354.73341342347 -24126.0658625139]  x3=[-2.1e-05 -3.12573992157971e-12 -11.1569792961398 -79.1361755515044;-2e-05 -3.12693823123776e-12 -11.1271448686892 -79.1403760100002;-1.9e-05 -3.12813609648814e-12 -11.0973088598231 -79.1445652208836;-1.8e-05 -3.12933351716063e-12 -11.067471273782 -79.1487431835592;-1.7e-05 -3.13053049308504e-12 -11.0376321148064 -79.1529098974333;-1.6e-05 -3.13172702409124e-12 -11.0077913871371 -79.1570653619137;-1.5e-05 -3.13292311000919e-12 -10.9779490950151 -79.1612095764097;-1.4e-05 -3.1341187506689e-12 -10.9481052426818 -79.1653425403324;-1.3e-05 -3.13531394590044e-12 -10.9182598343785 -79.1694642530944;-1.2e-05 -3.13650869553395e-12 -10.888412874347 -79.17357471411;-1.1e-05 -3.13770299939962e-12 -10.8585643668292 -79.1776739227948;-1e-05 -3.13889685732771e-12 -10.8287143160673 -79.1817618785664;-9e-06 -3.14009026914856e-12 -10.7988627263036 -79.1858385808438;-8e-06 -3.14128323469256e-12 -10.7690096017806 -79.1899040290475;-7e-06 -3.14247575379015e-12 -10.7391549467412 -79.1939582225998;-6e-06 -3.14366782627185e-12 -10.7092987654284 -79.1980011609244;-5e-06 -3.14485945196825e-12 -10.6794410620853 -79.2020328434469;-4e-06 -3.14605063070998e-12 -10.6495818409556 -79.2060532695941;-3e-06 -3.14724136232776e-12 -10.6197211062828 -79.2100624387947;-2e-06 -3.14843164665235e-12 -10.5898588623107 -79.214060350479;-1e-06 -3.14962148351458e-12 -10.5599951132835 -79.2180470040786]  x4=[-2.1e-05 -1.9203909728374e-12 -12.5606324026108 -78.9000787577024;-2e-05 -1.9195103512461e-12 -12.5308868818072 -78.9048083977175;-1.9e-05 -1.91862945684957e-12 -12.5011395800851 -78.9095268235996;-1.8e-05 -1.917748289773e-12 -12.4713905016723 -78.9142340346782;-1.7e-05 -1.91686685014164e-12 -12.4416396507968 -78.9189300302841;-1.6e-05 -1.91598513808074e-12 -12.4118870316868 -78.92361480975;-1.5e-05 -1.91510315371563e-12 -12.3821326485709 -78.9282883724102;-1.4e-05 -1.91422089717165e-12 -12.3523765056778 -78.9329507176004;-1.3e-05 -1.91333836857419e-12 -12.3226186072364 -78.9376018446579;-1.2e-05 -1.91245556804868e-12 -12.2928589574762 -78.9422417529218;-1.1e-05 -1.91157249572057e-12 -12.2630975606266 -78.9468704417325;-1e-05 -1.91068915171539e-12 -12.2333344209173 -78.9514879104323;-9e-06 -1.90980553615867e-12 -12.2035695425784 -78.9560941583649;-8e-06 -1.90892164917599e-12 -12.17380292984 -78.9606891848758;-7e-06 -1.90803749089296e-12 -12.1440345869328 -78.9652729893117;-6e-06 -1.90715306143526e-12 -12.1142645180874 -78.9698455710212;-5e-06 -1.90626836092858e-12 -12.0844927275349 -78.9744069293546;-4e-06 -1.90538338949865e-12 -12.0547192195065 -78.9789570636634;-3e-06 -1.90449814727125e-12 -12.0249439982336 -78.9834959733011;-2e-06 -1.90361263437218e-12 -11.995167067948 -78.9880236576225;-1e-06 -1.90272685092731e-12 -11.9653884328816 -78.9925401159843]  x5=2.03919101606495e-05  V1=ones(3,3)  V2=ones(3,3)  I1=ones(3,3)  I2=ones(3,3)  nHarmo=1  Measurements=None  Decoupling=off  VsMag0=0  VrMag0=0  VsAngle0=0  VrAngle0=0  IsMag0=0  IrMag0=0  IsAngle0=0  IrAngle0=0
      settings: LibrarySourceBlock=sps_lib/Power Grid Elements/Distributed Parameters Line
  Ground3 : spsGroundLib/Ground  LConnTagsString=a
  "Grounding Transformer " : spsGroundingTransformerLib/Grounding Transformer   UNITS=pu  NominalPower="[100e6   60]"  NominalVoltage=25e3  ZeroSequenceImpedance_pu=[0.025 0.75]  MagnetizationBranch_pu=[500 500]  ZeroSequenceImpedance_SI=[0.052083 589.05]  MagnetizationBranch_SI=[1041.7 3.927e+005]  Measurements=None
      settings: LibrarySourceBlock=|
      | sps_lib/Power Grid Elements/Grounding
      | Transformer
  A : PMIOPort  Side=Left
  B : PMIOPort  Port=2  Side=Left
  C : PMIOPort  Port=3  Side=Left
  connections:
  "3.3ohms "/RConn1 -- Ground3/LConn1
  120 kV / 25 kV 47 MVA/LConn1 -- 120kV 2500MVA/RConn1
  120 kV / 25 kV 47 MVA/LConn2 -- 120kV 2500MVA/RConn2
  120 kV / 25 kV 47 MVA/LConn3 -- 120kV 2500MVA/RConn3
  120 kV / 25 kV 47 MVA/RConn1 -- "Grounding Transformer "/LConn1 -- 14-km Feeder/RConn1 -- 30-MW 2-Mvar Load/LConn1
  120 kV / 25 kV 47 MVA/RConn2 -- "Grounding Transformer "/LConn2 -- 14-km Feeder/RConn2 -- 30-MW 2-Mvar Load/LConn2
  120 kV / 25 kV 47 MVA/RConn3 -- "Grounding Transformer "/LConn3 -- 14-km Feeder/RConn3 -- 30-MW 2-Mvar Load/LConn3
  5-km Feeder/RConn1 -- 14-km Feeder/LConn1 -- 2-MW Load/LConn1
  5-km Feeder/RConn2 -- 14-km Feeder/LConn2 -- 2-MW Load/LConn2
  5-km Feeder/RConn3 -- 14-km Feeder/LConn3 -- 2-MW Load/LConn3
  A/RConn1 -- 5-km Feeder/LConn1
  B/RConn1 -- 5-km Feeder/LConn2
  C/RConn1 -- 5-km Feeder/LConn3
  "Grounding Transformer "/RConn1 -- "3.3ohms "/LConn1

== system pso_mppt_grid_det/Efficiency ==
  Gain : Gain  Gain=100
  Product : Product  Inputs=/*
  Out1 : Outport  VectorParamsAs1DForOutWhenUnconnected=off
  wires:
  [P_B1_kW] -> Product/2
  Product/1 -> Gain/1
  [Pmean_PV] -> Product/1
  Gain/1 -> Out1/1

== system pso_mppt_grid_det/Irradiance Temp ==
  Demux : Demux  Tag=STV Demux  Outputs=2
      settings: DisplayOption=none
  FromWs : FromWorkspace  Tag=STV FromWs  VariableName=tuvar
      SigBuilderData=|
      | common.afterFinalStr = 'Extrapolate'
      | common.sampleTime = '0'
      | dataSet(1).timeRange = [0 2]
      | dataSet(1).name = 'Constant Irradiance'
      | dataSet(2).timeRange = [0 2]
      | dataSet(2).name = 'Step Irradiance'
      | dataSet(3).timeRange = [0 3]
      | dataSet(3).name = 'Ramp-up/down Irradiance'
      | sbobj.Groups(1).Name = 'Constant Irradiance'
      | sbobj.Groups(1).Signals(1).Name = 'Ir'
      | sbobj.Groups(1).Signals(1).XData = [0 2]
      | sbobj.Groups(1).Signals(1).YData = [1000 1000]
      | sbobj.Groups(1).Signals(2).Name = 'Temp'
      | sbobj.Groups(1).Signals(2).XData = [0 1 1 2]
      | sbobj.Groups(1).Signals(2).YData = [0 0 1 1]
      | sbobj.Groups(1).TimeRange = [0 2]
      | sbobj.Groups(2).Name = 'Step Irradiance'
      | sbobj.Groups(2).Signals(1).Name = 'Ir'
      | sbobj.Groups(2).Signals(1).XData = [0 0.252 0.252 2]
      | sbobj.Groups(2).Signals(1).YData = [600 600 1000 1000]
      | sbobj.Groups(2).Signals(2).Name = 'Temp'
      | sbobj.Groups(2).Signals(2).XData = [0 1 1 2]
      | sbobj.Groups(2).Signals(2).YData = [0 0 1 1]
      | sbobj.Groups(2).TimeRange = [0 2]
      | sbobj.Groups(3).Name = 'Ramp-up/down Irradiance'
      | sbobj.Groups(3).Signals(1).Name = 'Ir'
      | sbobj.Groups(3).Signals(1).XData = [0 0.6 1.1 1.2 1.7 3]
      | sbobj.Groups(3).Signals(1).YData = [1000 1000 250 250 1000 1000]
      | sbobj.Groups(3).Signals(2).Name = 'Temp'
      | sbobj.Groups(3).Signals(2).XData = [0 2 2.1 3]
      | sbobj.Groups(3).Signals(2).YData = [25 25 50 50]
      | sbobj.Groups(3).TimeRange = [0 3]
  Ir : Outport  Tag=STV Outport  VectorParamsAs1DForOutWhenUnconnected=off
  Temp : Outport  Tag=STV Outport  Port=2  VectorParamsAs1DForOutWhenUnconnected=off
  wires:
  Demux/1 -> Ir/1
  FromWs/1 -> Demux/1
  Demux/2 -> Temp/1

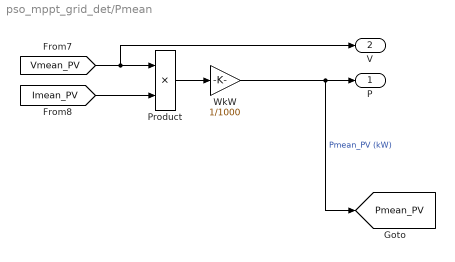
== system pso_mppt_grid_det/Pmean ==
  Product : Product  RndMeth=Zero
  WkW : Gain  Gain=1/1000
  P : Outport  VectorParamsAs1DForOutWhenUnconnected=off
  V : Outport  Port=2  VectorParamsAs1DForOutWhenUnconnected=off
  tag scope: Pmean_PV=global
  wires:
  [Vmean_PV] -> Product/1, V/1
  Product/1 -> WkW/1
  [Imean_PV] -> Product/2
  WkW/1 -> [Pmean_PV], P/1  "Pmean_PV (kW)"

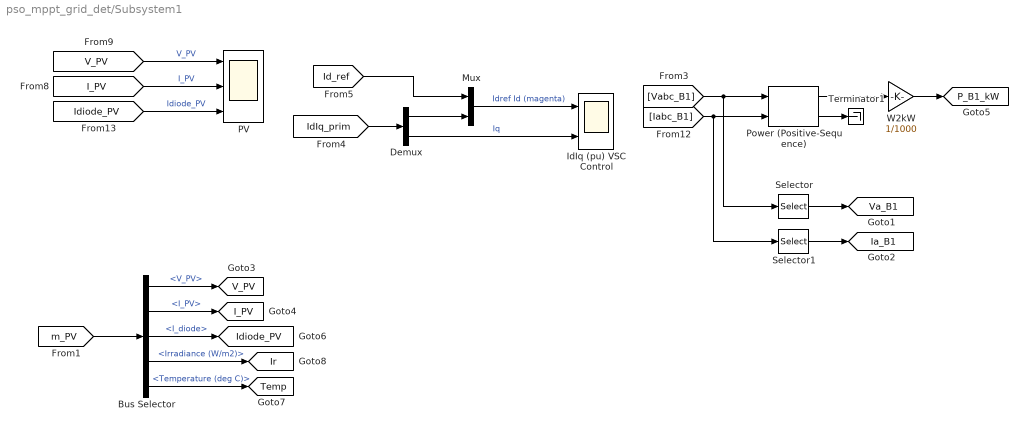
== system pso_mppt_grid_det/Subsystem1 ==
  Bus Selector : BusSelector  OutputSignals=V_PV,I_PV,I_diode,Irradiance (W/m2),Temperature (deg C)
  Demux : Demux  Outputs=2
  IdIq (pu) VSC Control : Scope  NumInputPorts=2
  Mux : Mux  Inputs=2
  PV : Scope  NumInputPorts=3
  Power (Positive-Sequence) : spsPowerPositiveSequenceLib/Power (Positive-Sequence)  Freq=60  Vinit=[0, 0]  Iinit=[0, 0]  Ts=Ts_Control
      settings: LibrarySourceBlock=|
      | sps_lib/Sensors and Measurements/Power
      | (Positive-Sequence)
  Selector : Selector  InputPortWidth=3  IndexOptions=Index vector (dialog)  Indices=[1]  OutputSizes=1
  Selector1 : Selector  InputPortWidth=3  IndexOptions=Index vector (dialog)  Indices=[1]  OutputSizes=1
  Terminator1 : Terminator
  W2kW : Gain  Gain=1/1000
  tag scope: I_PV=global, Ia_B1=global, Idiode_PV=global, Ir=global, P_B1_kW=global, Temp=global, V_PV=global, Va_B1=global
  wires:
  [Vabc_B1] -> Power (Positive-Sequence)/1, Selector/1
  [Iabc_B1] -> Power (Positive-Sequence)/2, Selector1/1
  Power (Positive-Sequence)/1 -> W2kW/1
  [IdIq_prim] -> Demux/1
  [Id_ref] -> Mux/1
  Demux/1 -> Mux/2
  Mux/1 -> IdIq (pu) VSC Control/1  "Idref Id (magenta)"
  Demux/2 -> IdIq (pu) VSC Control/2  "Iq"
  Selector/1 -> [Va_B1]
  Selector1/1 -> [Ia_B1]
  [V_PV] -> PV/1  "V_PV"
  [I_PV] -> PV/2  "I_PV"
  [Idiode_PV] -> PV/3  "Idiode_PV"
  W2kW/1 -> [P_B1_kW]
  [m_PV] -> Bus Selector/1
  Bus Selector/1 -> [V_PV]  "<V_PV>"
  Bus Selector/2 -> [I_PV]  "<I_PV>"
  Bus Selector/4 -> [Ir]  "<Irradiance (W/m2)>"
  Bus Selector/3 -> [Idiode_PV]  "<I_diode>"
  Bus Selector/5 -> [Temp]  "<Temperature (deg C)>"
  Power (Positive-Sequence)/2 -> Terminator1/1

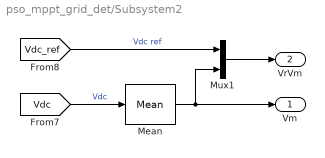
== system pso_mppt_grid_det/Subsystem2 ==
  Mean : spsMeanLib/Mean  Freq=60  Vinit=0  Ts=Ts_Control
  Mux1 : Mux  Inputs=2
  Vm : Outport  VectorParamsAs1DForOutWhenUnconnected=off
  VrVm : Outport  Port=2  VectorParamsAs1DForOutWhenUnconnected=off
  wires:
  [Vdc_ref] -> Mux1/1  "Vdc ref"
  [Vdc] -> Mean/1  "Vdc"
  Mux1/1 -> VrVm/1
  Mean/1 -> Mux1/2, Vm/1

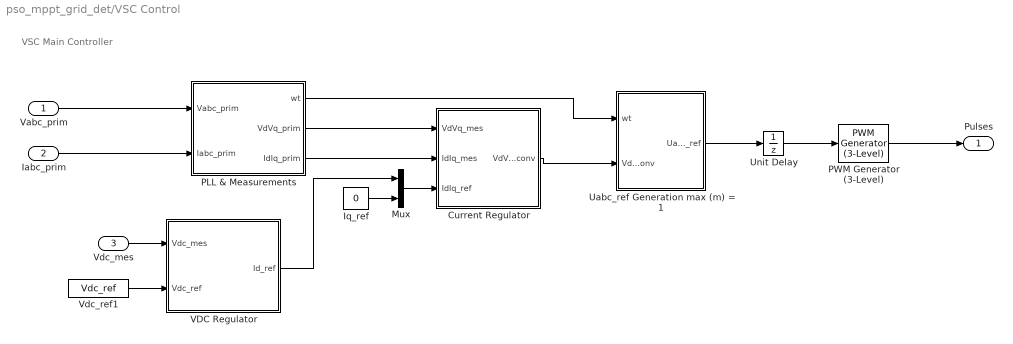
== system pso_mppt_grid_det/VSC Control ==
  note: VSC Main Controller
  Vabc_prim : Inport  PortDimensions=3
  Iabc_prim : Inport  Port=2  PortDimensions=3
  Vdc_mes : Inport  Port=3  PortDimensions=1
  Current Regulator : Subsystem
  Iq_ref : Constant  Value=0
  Mux : Mux  Inputs=2
  PLL & Measurements : Subsystem
  PWM Generator (3-Level) : spsPWMGenerator3LevelLib/PWM Generator (3-Level)  ModulatorType=Three-phase bridge (12 pulses)  ModulatorMode=Unsynchronized  nF=27  Fc=33*60  ModulatingSignals=off  m=0.8  Freq=60  Phase=0  Ts=Ts_Power
      settings: LibrarySourceBlock=|
      | sps_lib/Power Electronics/Power Electronics Control/PWM Generator
      | (3-Level)
  Uabc_ref Generation max (m) = 1 : Subsystem
  Unit Delay : UnitDelay  SampleTime=Ts_Control  HasFrameUpgradeWarning=on
  VDC Regulator : Subsystem
  Vdc_ref1 : Constant  Value=Vdc_ref
  Pulses : Outport  VectorParamsAs1DForOutWhenUnconnected=off
  wires:
  VDC Regulator/1(Id_ref) -> Mux/1
  PLL & Measurements/1(wt) -> Uabc_ref Generation max (m) = 1/1(wt)
  Current Regulator/1(VdVq_conv) -> Uabc_ref Generation max (m) = 1/2(VdVq_conv)
  Iq_ref/1 -> Mux/2
  Mux/1 -> Current Regulator/3(IdIq_ref)
  PLL & Measurements/3(IdIq_prim) -> Current Regulator/2(IdIq_mes)
  PLL & Measurements/2(VdVq_prim) -> Current Regulator/1(VdVq_mes)
  Vdc_mes/1 -> VDC Regulator/1(Vdc_mes)
  Vabc_prim/1 -> PLL & Measurements/1(Vabc_prim)
  Iabc_prim/1 -> PLL & Measurements/2(Iabc_prim)
  Unit Delay/1 -> PWM Generator (3-Level)/1
  PWM Generator (3-Level)/1 -> Pulses/1
  Uabc_ref Generation max (m) = 1/1(Uabc_ref) -> Unit Delay/1
  Vdc_ref1/1 -> VDC Regulator/2(Vdc_ref)

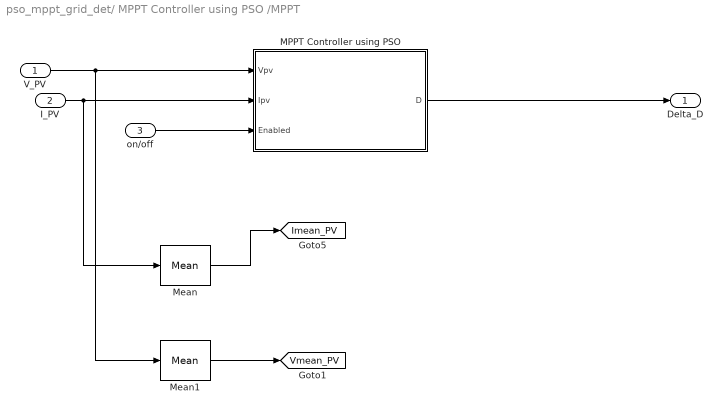
== system pso_mppt_grid_det/ MPPT Controller using PSO /MPPT ==
  V_PV : Inport
  I_PV : Inport  Port=2
  on/off : Inport  Port=3
  "MPPT Controller using PSO " : MATLAB Function  TreatAsAtomicUnit=on
  Mean : spsMeanLib/Mean  Freq=1/T_MPPT  Vinit=0  Ts=Ts_Control
  Mean1 : spsMeanLib/Mean  Freq=1/T_MPPT  Vinit=0  Ts=Ts_Control
  Delta_D : Outport  VectorParamsAs1DForOutWhenUnconnected=off
  tag scope: Imean_PV=global, Vmean_PV=global
  wires:
  Mean1/1 -> [Vmean_PV]
  Mean/1 -> [Imean_PV]
  V_PV/1 -> Mean1/1, "MPPT Controller using PSO "/1(Vpv)
  I_PV/1 -> Mean/1, "MPPT Controller using PSO "/2(Ipv)
  on/off/1 -> "MPPT Controller using PSO "/3(Enabled)
  "MPPT Controller using PSO "/1(D) -> Delta_D/1

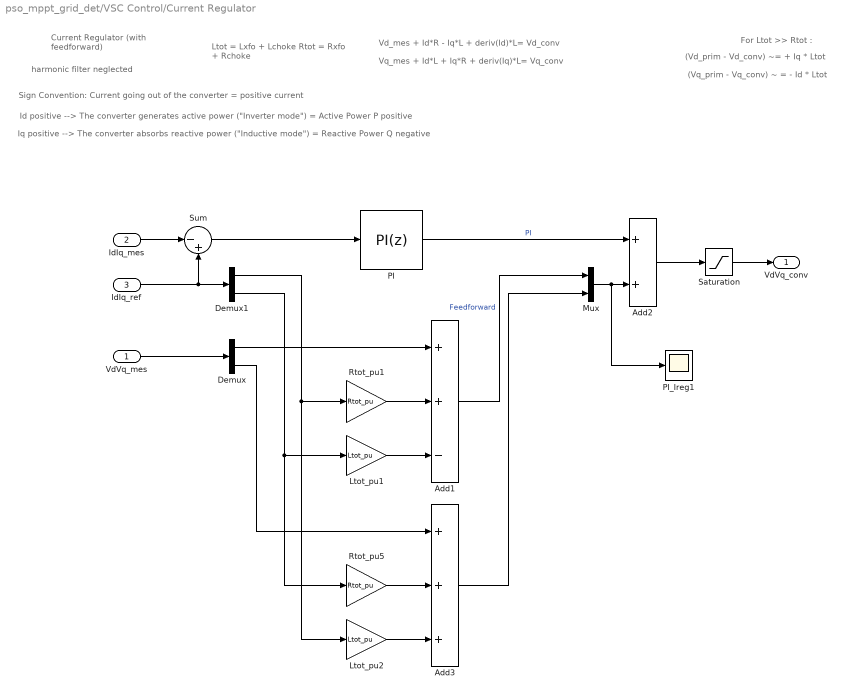
== system pso_mppt_grid_det/VSC Control/Current Regulator ==
  note: harmonic filter neglected
  note: Vd_mes + Id*R - Iq*L + deriv(Id)*L= Vd_conv
  note: Vq_mes + Id*L + Iq*R + deriv(Iq)*L= Vq_conv
  note: Current Regulator
      | (with feedforward)
  note: Sign Convention: Current going out of the converter = positive current
  note: Iq positive --> The converter absorbs reactive power ("Inductive mode") = Reactive Power Q negative
  note: Id positive --> The converter generates active power ("Inverter mode") = Active Power P positive
  note: Ltot = Lxfo + Lchoke
      | Rtot = Rxfo + Rchoke
  note: (Vd_prim - Vd_conv) ~= + Iq * Ltot
  note: (Vq_prim - Vq_conv) ~ = - Id * Ltot
  note: For Ltot >> Rtot :
  VdVq_mes : Inport  PortDimensions=2
  IdIq_mes : Inport  Port=2  PortDimensions=2
  IdIq_ref : Inport  Port=3  PortDimensions=2
  Add1 : Sum  Inputs=++-
  Add2 : Sum
  Add3 : Sum  Inputs=+++
  Demux : Demux  Outputs=2
  Demux1 : Demux  Outputs=2
  Ltot_pu1 : Gain  Gain=Ltot_pu  SaturateOnIntegerOverflow=on  OutDataTypeStr=Inherit: Same as input  ParamDataTypeStr=Inherit: Same as input
  Ltot_pu2 : Gain  Gain=Ltot_pu  SaturateOnIntegerOverflow=on  OutDataTypeStr=Inherit: Same as input  ParamDataTypeStr=Inherit: Same as input
  Mux : Mux  Inputs=2
  PI : slpidlib/PID Controller  Controller=PI  Form=Parallel  TimeDomain=Discrete-time  UseExternalTs=off  SampleTime=Ts  IntegratorMethod=Forward Euler  FilterMethod=Forward Euler  ControllerParametersSource=internal  P=Kp_Ireg  I=Ki_Ireg  UseKiTs=off  D=0  UseExternalDerivativeSource=off  N=100  UseFilter=on  TunerSelectOption=Transfer Function Based (PID Tuner App)  InitialConditionSource=internal  InitialConditionForIntegrator=0  InitialConditionForFilter=0  DifferentiatorICPrevScaledInput=0  ExternalReset=none  TrackingMode=off  Kt=1  LimitOutput=on  SatLimitsSource=internal  UpperSaturationLimit=2  LowerSaturationLimit=-2  LinearizeAsGain=off  AntiWindupMode=none  Kb=1  LimitIntegrator=off  UpperIntegratorSaturationLimit=inf  LowerIntegratorSaturationLimit=-inf  POutMin=[]  POutMax=[]  IOutMin=[]  IOutMax=[]  DOutMin=[]  DOutMax=[]  NOutMin=[]  NOutMax=[]  SumOutMin=[]  SumOutMax=[]  SaturationOutMin=[]  SaturationOutMax=[]  PParamMin=[]  PParamMax=[]  IParamMin=[]  IParamMax=[]  DParamMin=[]  DParamMax=[]  NParamMin=[]  NParamMax=[]  KbParamMin=[]  KbParamMax=[]  KtParamMin=[]  KtParamMax=[]  KbOutMin=[]  KbOutMax=[]  KtOutMin=[]  KtOutMax=[]  IntegratorOutMin=[]  IntegratorOutMax=[]  FilterOutMin=[]  FilterOutMax=[]  SumI1OutMin=[]  SumI1OutMax=[]  SumI2OutMin=[]  SumI2OutMax=[]  SumI3OutMin=[]  SumI3OutMax=[]  SumI4OutMin=[]  SumI4OutMax=[]  SumDOutMin=[]  SumDOutMax=[]  DifferentiatorOutMin=[]  DifferentiatorOutMax=[]  FilterDiffOutCoefMin=[]  FilterDiffOutCoefMax=[]  ReciprocalOutMin=[]  ReciprocalOutMax=[]  SumDenOutMin=[]  SumDenOutMax=[]  SumNumOutMin=[]  SumNumOutMax=[]  DivideOutMin=[]  DivideOutMax=[]  UdiffTsProdOutMin=[]  UdiffTsProdOutMax=[]  NTsProdOutMin=[]  NTsProdOutMax=[]  UintegralTsProdOutMin=[]  UintegralTsProdOutMax=[]  UngainTsProdOutMin=[]  UngainTsProdOutMax=[]  ClampingZeroOutDataTypeStr=Inherit: Inherit via back propagation  ClampingZeroOutMin=[]  ClampingZeroOutMax=[]  FilterDenConstantOutDataTypeStr=Inherit: Inherit via back propagation  FilterDenConstantOutMin=[]  FilterDenConstantOutMax=[]  PCopyOutDataTypeStr=Inherit: Inherit via back propagation  PCopyOutMin=[]  PCopyOutMax=[]  NCopyOutDataTypeStr=Inherit: Inherit via back propagation  NCopyOutMin=[]  NCopyOutMax=[]  IntegratorContinuousStateAttributes=''  IntegratorStateMustResolveToSignalObject=off  IntegratorRTWStateStorageClass=Auto  FilterContinuousStateAttributes=''  FilterStateMustResolveToSignalObject=off  FilterRTWStateStorageClass=Auto  ParallelPVariant=InternalParameters  IdealPVariant=Disabled  IVariant=InternalParameters  DVariant=Disabled  IntegratorVariant=Discrete  SatVariant=Enabled  AWVariant=Passthrough  PCopyVariant=Disabled  TRVariant=Disabled  FdbkBlocksVariant=Forward  IdealPFdbkVariant=Disabled  SatFdbkVariant=Disabled  DerivativeFilterVariant=Disabled  NVariant=Disabled  NCopyVariant=Disabled_SignalSpec  FilterICVariant=Disabled  IntegratorICVariant=InternalICs  ExternalResetVariant=Disabled  TRSumVariant=Passthrough  SumFdbkVariant=Disabled  SumVariant=Sum_PI  TsampFilterVariant=InternalTs  TsampNgainVariant=Passthrough  TsampIntegralVariant=Disabled_SignalSpec  ExternalSaturationOutDataTypeStr=Inherit: Same as second input  DerivativeSourceVariant=Disabled
  PI_Ireg1 : Scope
  Rtot_pu1 : Gain  Gain=Rtot_pu  SaturateOnIntegerOverflow=on  OutDataTypeStr=Inherit: Same as input  ParamDataTypeStr=Inherit: Same as input
  Rtot_pu5 : Gain  Gain=Rtot_pu  SaturateOnIntegerOverflow=on  OutDataTypeStr=Inherit: Same as input  ParamDataTypeStr=Inherit: Same as input
  Saturation : Saturate  UpperLimit=2  LowerLimit=-2
  Sum : Sum  Inputs=|-+
  VdVq_conv : Outport  VectorParamsAs1DForOutWhenUnconnected=off
  wires:
  Mux/1 -> PI_Ireg1/1, Add2/2
  PI/1 -> Add2/1  "PI"
  Sum/1 -> PI/1
  IdIq_ref/1 -> Sum/2, Demux1/1
  IdIq_mes/1 -> Sum/1
  Add2/1 -> Saturation/1
  Saturation/1 -> VdVq_conv/1
  VdVq_mes/1 -> Demux/1
  Demux/1 -> Add1/1
  Rtot_pu1/1 -> Add1/2
  Demux1/1 -> Rtot_pu1/1, Ltot_pu2/1
  Ltot_pu1/1 -> Add1/3
  Demux1/2 -> Ltot_pu1/1, Rtot_pu5/1
  Rtot_pu5/1 -> Add3/2
  Ltot_pu2/1 -> Add3/3
  Add1/1 -> Mux/1  "Feedforward"
  Demux/2 -> Add3/1
  Add3/1 -> Mux/2
